simulink library "LibControllers"  (R2015b)
settings: Solver=ode45  SolverMode=SingleTasking  StartTime=0.0  StopTime=10.0  RelTol=1e-3
undefined symbols (not defined in the file or in its folder): accelCanon, adjustCoefficients, bw, depth, DiscIntNeverNeededParam, displCanon, forget, freq, initDispl, jerkCanon, kd, kdp, kf, ki, kp, maxAuthority, maxForce, nominFlow, p, R, ratedFlow, S, samplePeriod, T, velocCanon
undefined symbols (not defined in the file): fbkgen, fdp, fmax, fmin, gainRatio, interval, lagFreq, lagPhase, leadFreq, leadPhase, order, refabort, refgen, refsmooth, supplyPress, vmax, vmin
libraries: LibControllers x43, simulink x1
(part 2 of 2)

== system LibControllers/forward euler integrator with clipping ==
  inp : Inport
  Saturation : Saturate  UpperLimit=maxOutput  LowerLimit=minOutput
  Sum1 : Sum  Inputs=|++  SaturateOnIntegerOverflow=on  InputSameDT=on  OutDataTypeStr=Inherit: Same as first input
  T : Gain  Gain=samplePeriod
  Unit Delay : UnitDelay  SampleTime=-1
  Unit Delay1 : UnitDelay  InitialCondition=initialCondition  SampleTime=-1
  out : Outport
  wires:
  Saturation/1 -> Unit Delay1/1, out/1
  inp/1 -> Unit Delay/1
  Unit Delay/1 -> T/1
  Unit Delay1/1 -> Sum1/2
  Sum1/1 -> Saturation/1
  T/1 -> Sum1/1

== system LibControllers/generic controller ==
  cmd : Inport
  fbk : Inport  Port=2
  Sum : Sum  Inputs=|+-
  feedback polynomial : DiscreteFir  Coefficients=adjustCoefficients(S)  AccumDataTypeStr=Inherit: Same as product output
  feedforward polynomial : DiscreteFir  Coefficients=(T).'  AccumDataTypeStr=Inherit: Same as product output
  output scaling : Gain  Gain=k
  regression polynomial : DiscreteFilter  Denominator=R
  out : Outport
  wires:
  regression polynomial/1 -> output scaling/1
  Sum/1 -> regression polynomial/1
  feedforward polynomial/1 -> Sum/1
  feedback polynomial/1 -> Sum/2
  cmd/1 -> feedforward polynomial/1
  fbk/1 -> feedback polynomial/1
  output scaling/1 -> out/1

== system LibControllers/lag compensator ==
  inp : Inport
  Discrete Filter : DiscreteFilter  Numerator=b  Denominator=a
  out : Outport
  wires:
  Discrete Filter/1 -> out/1
  inp/1 -> Discrete Filter/1

== system LibControllers/lead compensator ==
  inp : Inport
  Discrete Filter : DiscreteFilter  Numerator=b  Denominator=a
  out : Outport
  wires:
  Discrete Filter/1 -> out/1
  inp/1 -> Discrete Filter/1

== system LibControllers/max//min cyclic fg ==
  Sum : Sum  Inputs=|++
  mean level : Constant  Value=mean
  shape : Constant  Value=shape
  sine wave : Sin  Amplitude=ampl  Frequency=2 * pi * freq  Phase=phase * pi/180  SampleTime=sourceSamplePeriod
  square wave : Subsystem  mask(Repeating table){ampl=ampl, freq=freq, phase=phase, samplePeriod=samplePeriod}
      mask prompts: ampl "Amplitude"; freq "Frequency (Hz)"; phase "Phase (deg)"; samplePeriod "Sample period (sec)"
      mask help: Output a repeating sequence of numbers specified in a table of time-value pairs. Values of time should be monotonically increasing.
      mask init:
      | % phase must be positive
      | while phase < 0
      | 	phase = phase + 360;
      | end
      mask Help: Repeats cycle given in table. Time values should be monotonically increasing.
  triangle wave : Subsystem  mask(Repeating table){ampl=ampl, freq=freq, phase=phase, samplePeriod=samplePeriod}
      mask prompts: ampl "Amplitude"; freq "Frequency (Hz)"; phase "Phase (deg)"; samplePeriod "Sample period (sec)"
      mask help: Output a repeating sequence of numbers specified in a table of time-value pairs. Values of time should be monotonically increasing.
      mask init:
      | % phase must be positive
      | while phase < 0
      | 	phase = phase + 360;
      | end
      mask Help: Repeats cycle given in table. Time values should be monotonically increasing.
  waveform selector : MultiPortSwitch
  out : Outport
  wires:
  mean level/1 -> Sum/2
  Sum/1 -> out/1
  shape/1 -> waveform selector/1
  square wave/1(out) -> waveform selector/2
  triangle wave/1(out) -> waveform selector/3
  sine wave/1 -> waveform selector/4
  waveform selector/1 -> Sum/1

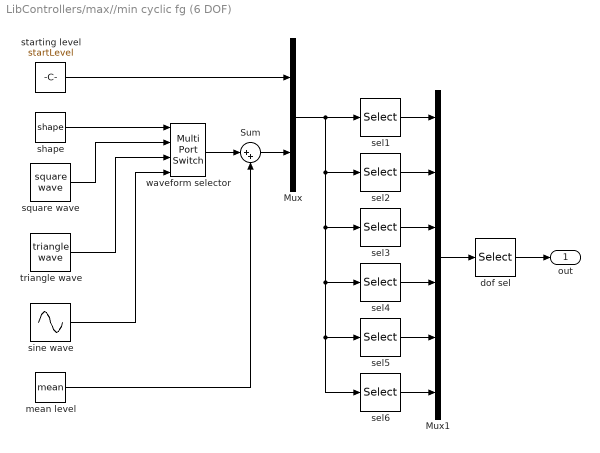
== system LibControllers/max//min cyclic fg (6 DOF) ==
  Mux : Mux  Inputs=2
  Mux1 : Mux  Inputs=6
  Sum : Sum  Inputs=|++
  dof sel : Selector  IndexOptions=Index vector (dialog)  Indices=dof  OutputSizes=1
  mean level : Constant  Value=mean
  sel1 : Selector  InputPortWidth=2  IndexOptions=Index vector (dialog)  Indices=(id==1)+1  OutputSizes=1
  sel2 : Selector  InputPortWidth=2  IndexOptions=Index vector (dialog)  Indices=(id==2)+1  OutputSizes=1
  sel3 : Selector  InputPortWidth=2  IndexOptions=Index vector (dialog)  Indices=(id==3)+1  OutputSizes=1
  sel4 : Selector  InputPortWidth=2  IndexOptions=Index vector (dialog)  Indices=(id==4)+1  OutputSizes=1
  sel5 : Selector  InputPortWidth=2  IndexOptions=Index vector (dialog)  Indices=(id==5)+1  OutputSizes=1
  sel6 : Selector  InputPortWidth=2  IndexOptions=Index vector (dialog)  Indices=(id==6)+1  OutputSizes=1
  shape : Constant  Value=shape
  sine wave : Sin  Amplitude=ampl  Frequency=2 * pi * freq  Phase=phase * pi/180  SampleTime=sourceSamplePeriod
  square wave : LibControllers/cyclic fg/square wave  SystemSampleTime=-1  ampl=ampl  freq=freq  phase=phase  samplePeriod=samplePeriod
  starting level : Constant  Value=startLevel
  triangle wave : LibControllers/cyclic fg/triangle wave  SystemSampleTime=-1  ampl=ampl  freq=freq  phase=phase  samplePeriod=samplePeriod
  waveform selector : MultiPortSwitch
  out : Outport
  wires:
  Sum/1 -> Mux/2
  waveform selector/1 -> Sum/1
  Mux1/1 -> dof sel/1
  mean level/1 -> Sum/2
  starting level/1 -> Mux/1
  sel1/1 -> Mux1/1
  sel2/1 -> Mux1/2
  sel3/1 -> Mux1/3
  sel4/1 -> Mux1/4
  sel5/1 -> Mux1/5
  sel6/1 -> Mux1/6
  Mux/1 -> sel2/1, sel3/1, sel4/1, sel5/1, sel6/1, sel1/1
  sine wave/1 -> waveform selector/4
  triangle wave/1 -> waveform selector/3
  square wave/1 -> waveform selector/2
  shape/1 -> waveform selector/1
  dof sel/1 -> out/1

== system LibControllers/notch filter ==
  inp : Inport
  Discrete Filter : DiscreteFilter  Numerator=b  Denominator=a
  out : Outport
  wires:
  Discrete Filter/1 -> out/1
  inp/1 -> Discrete Filter/1

== system LibControllers/pi controller ==
  cmd : Inport
  fbk : Inport  Port=2
  Sum : Sum  Inputs=|+-
  Sum1 : Sum  Inputs=|++
  egu to volts : Gain  Gain=10/maxUnits
  integrator with clipping : LibControllers/backward euler integrator with clipping  SystemSampleTime=-1  initialCondition=0  maxOutput=0.01*maxAuthority*maxUnits  minOutput=-0.01*maxAuthority*maxUnits  samplePeriod=samplePeriod
  ki : Gain  Gain=ki
  kp : Gain  Gain=kp
  out : Outport
  wires:
  Sum/1 -> kp/1, integrator with clipping/1
  cmd/1 -> Sum/1
  fbk/1 -> Sum/2
  kp/1 -> Sum1/1
  ki/1 -> Sum1/2
  integrator with clipping/1 -> ki/1
  Sum1/1 -> egu to volts/1
  egu to volts/1 -> out/1

== system LibControllers/pid controller ==
  cmd : Inport
  fbk : Inport  Port=2
  Sum : Sum  Inputs=|+-
  Sum1 : Sum  Inputs=++-
  Sum2 : Sum  Inputs=|++
  egu to volts : Gain  Gain=10/maxUnits
  fb break filter : Subsystem  mask(First-Order Lowpass Filter){freq=bw, samplePeriod=samplePeriod}
      mask prompts: freq "Cutoff frequency (Hz)"; samplePeriod "Sample period (sec)"
      mask init:
      | bwt = freq * samplePeriod;
      | if (bwt > 0.5*0.95) 
      | 	a = [1];
      | 	b = [1];
      | else	% first-order
      | 	c	 = 1 / tan(pi * bwt);
      | 	bwt2 = 1.0 / (pi * c);	% prewarp
      | 	a    = [1 -exp(-2*pi*bwt2)];
      | 	b	 = [1] * sum(a);
      | end
  fb derivative : LibControllers/euler derivative  SystemSampleTime=-1  initialCondition=0  samplePeriod=samplePeriod
  ff break filter : Subsystem  mask(First-Order Lowpass Filter){freq=bw, samplePeriod=samplePeriod}
      mask prompts: freq "Cutoff frequency (Hz)"; samplePeriod "Sample period (sec)"
      mask init:
      | bwt = freq * samplePeriod;
      | if (bwt > 0.5*0.95) 
      | 	a = [1];
      | 	b = [1];
      | else	% first-order
      | 	c	 = 1 / tan(pi * bwt);
      | 	bwt2 = 1.0 / (pi * c);	% prewarp
      | 	a    = [1 -exp(-2*pi*bwt2)];
      | 	b	 = [1] * sum(a);
      | end
  ff derivative : LibControllers/euler derivative  SystemSampleTime=-1  initialCondition=0  samplePeriod=samplePeriod
  integrator with clipping : LibControllers/backward euler integrator with clipping  SystemSampleTime=-1  initialCondition=0  maxOutput=0.01*maxAuthority*maxUnits  minOutput=-0.01*maxAuthority*maxUnits  samplePeriod=samplePeriod
  ki : Gain  Gain=ki
  ki1 : Gain  Gain=kd
  kp : Gain  Gain=kp
  kp1 : Gain  Gain=kf
  second-order butterworth lowpass filter : LibControllers/second-order butterworth lowpass filter  SystemSampleTime=-1  freq=bw  samplePeriod=samplePeriod
  out : Outport
  wires:
  egu to volts/1 -> out/1
  integrator with clipping/1 -> ki/1
  kp/1 -> Sum1/2
  kp1/1 -> Sum1/1
  fb break filter/1(out) -> ki1/1
  ff break filter/1(out) -> kp1/1
  second-order butterworth lowpass filter/1 -> Sum2/1
  Sum1/1 -> second-order butterworth lowpass filter/1
  ff derivative/1 -> ff break filter/1(inp)
  fbk/1 -> Sum/2, fb derivative/1
  cmd/1 -> Sum/1, ff derivative/1
  Sum/1 -> kp/1, integrator with clipping/1
  fb derivative/1 -> fb break filter/1(inp)
  ki1/1 -> Sum1/3
  Sum2/1 -> egu to volts/1
  ki/1 -> Sum2/2

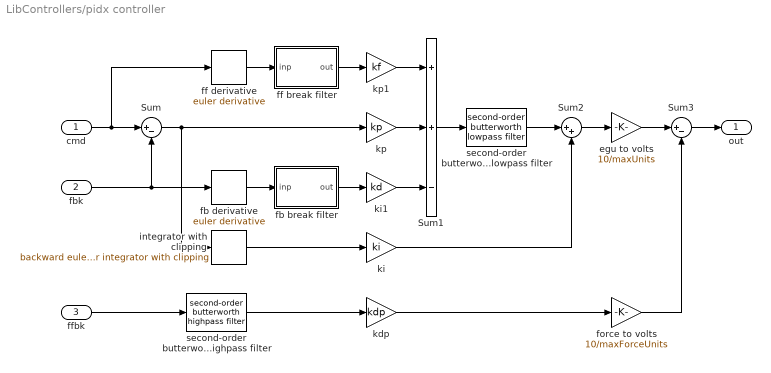
== system LibControllers/pidx controller ==
  cmd : Inport
  fbk : Inport  Port=2
  ffbk : Inport  Port=3
  Sum : Sum  Inputs=|+-
  Sum1 : Sum  Inputs=++-
  Sum2 : Sum  Inputs=|++
  Sum3 : Sum  Inputs=|+-
  egu to volts : Gain  Gain=10/maxUnits
  fb break filter : Subsystem  mask(First-Order Lowpass Filter){freq=bw, samplePeriod=samplePeriod}
      mask prompts: freq "Cutoff frequency (Hz)"; samplePeriod "Sample period (sec)"
      mask init:
      | bwt = freq * samplePeriod;
      | if (bwt > 0.5*0.95) 
      | 	a = [1];
      | 	b = [1];
      | else	% first-order
      | 	c	 = 1 / tan(pi * bwt);
      | 	bwt2 = 1.0 / (pi * c);	% prewarp
      | 	a    = [1 -exp(-2*pi*bwt2)];
      | 	b	 = [1] * sum(a);
      | end
  fb derivative : LibControllers/euler derivative  SystemSampleTime=-1  initialCondition=0  samplePeriod=samplePeriod
  ff break filter : Subsystem  mask(First-Order Lowpass Filter){freq=bw, samplePeriod=samplePeriod}
      mask prompts: freq "Cutoff frequency (Hz)"; samplePeriod "Sample period (sec)"
      mask init:
      | bwt = freq * samplePeriod;
      | if (bwt > 0.5*0.95) 
      | 	a = [1];
      | 	b = [1];
      | else	% first-order
      | 	c	 = 1 / tan(pi * bwt);
      | 	bwt2 = 1.0 / (pi * c);	% prewarp
      | 	a    = [1 -exp(-2*pi*bwt2)];
      | 	b	 = [1] * sum(a);
      | end
  ff derivative : LibControllers/euler derivative  SystemSampleTime=-1  initialCondition=0  samplePeriod=samplePeriod
  force to volts : Gain  Gain=10/maxForceUnits
  integrator with clipping : LibControllers/backward euler integrator with clipping  SystemSampleTime=-1  initialCondition=0  maxOutput=0.01*maxAuthority*maxUnits  minOutput=-0.01*maxAuthority*maxUnits  samplePeriod=samplePeriod
  kdp : Gain  Gain=kdp
  ki : Gain  Gain=ki
  ki1 : Gain  Gain=kd
  kp : Gain  Gain=kp
  kp1 : Gain  Gain=kf
  second-order butterworth highpass filter : LibControllers/second-order butterworth highpass filter  SystemSampleTime=-1  freq=fdp  samplePeriod=samplePeriod
  second-order butterworth lowpass filter : LibControllers/second-order butterworth lowpass filter  SystemSampleTime=-1  freq=bw  samplePeriod=samplePeriod
  out : Outport
  wires:
  ki/1 -> Sum2/2
  kdp/1 -> force to volts/1
  integrator with clipping/1 -> ki/1
  kp/1 -> Sum1/2
  kp1/1 -> Sum1/1
  fb break filter/1(out) -> ki1/1
  ff break filter/1(out) -> kp1/1
  second-order butterworth highpass filter/1 -> kdp/1
  second-order butterworth lowpass filter/1 -> Sum2/1
  Sum1/1 -> second-order butterworth lowpass filter/1
  ff derivative/1 -> ff break filter/1(inp)
  ffbk/1 -> second-order butterworth highpass filter/1
  fbk/1 -> Sum/2, fb derivative/1
  cmd/1 -> Sum/1, ff derivative/1
  Sum/1 -> kp/1, integrator with clipping/1
  fb derivative/1 -> fb break filter/1(inp)
  ki1/1 -> Sum1/3
  Sum3/1 -> out/1
  Sum2/1 -> egu to volts/1
  egu to volts/1 -> Sum3/1
  force to volts/1 -> Sum3/2

== system LibControllers/power observer ==
  veloc : Inport
  force : Inport  Port=2
  force polarity switch : Switch
  max force : Constant  Value=abs(max(fmax, eps))
  max veloc : Constant  Value=abs(max(vmax, eps))
  min force : Constant  Value=abs(min(fmin, eps))
  min veloc : Constant  Value=abs(min(vmin, eps))
  neg scale : Gain  Gain=100 / sqrt(2)
  normalization : Product  Inputs=*/
  normalization factor : Product  RndMeth=Zero
  pos scale : Gain  Gain=100 * 2 * sqrt(2)
  power calculation : Product  RndMeth=Zero
  power polarity switch : Switch
  velocity polarity switch : Switch
  power : Outport
  wires:
  veloc/1 -> power calculation/1, velocity polarity switch/2
  force/1 -> power calculation/2, force polarity switch/2
  power calculation/1 -> normalization/1
  min veloc/1 -> velocity polarity switch/3
  max veloc/1 -> velocity polarity switch/1
  max force/1 -> force polarity switch/1
  min force/1 -> force polarity switch/3
  velocity polarity switch/1 -> normalization factor/1
  force polarity switch/1 -> normalization factor/2
  normalization factor/1 -> normalization/2
  power polarity switch/1 -> power/1
  normalization/1 -> pos scale/1, power polarity switch/2, neg scale/1
  pos scale/1 -> power polarity switch/1
  neg scale/1 -> power polarity switch/3

== system LibControllers/ramp fg ==
  integrator with clipping : LibControllers/forward euler integrator with clipping  SystemSampleTime=-1  initialCondition=startLevel  maxOutput=max(startLevel, endLevel)  minOutput=min(startLevel, endLevel)  samplePeriod=samplePeriod
  ramp rate : Constant  Value=(endLevel - startLevel) / max(interval, samplePeriod)
  out : Outport
  wires:
  ramp rate/1 -> integrator with clipping/1
  integrator with clipping/1 -> out/1

== system LibControllers/rand fg ==
  Product : Product  RndMeth=Zero
  biquad group 1 : Subsystem  mask(Discrete Filter Group of Five Biquads){sos=sos(1:5,:)}
      mask prompts: sos "Second-order sections"
  biquad group 2 : Subsystem  mask(Discrete Filter Group of Five Biquads){sos=sos(6:10,:)}
      mask prompts: sos "Second-order sections"
  biquad group 3 : Subsystem  mask(Discrete Filter Group of Five Biquads){sos=sos(11:15,:)}
      mask prompts: sos "Second-order sections"
  gain : Gain  Gain=g
  span fg : LibControllers/ramp fg  SystemSampleTime=-1  startLevel=0  endLevel=1  interval=spanInterval  samplePeriod=samplePeriod
  uniform rand : UniformRandomNumber  Minimum=-peakAmpl  Maximum=peakAmpl  Seed=seed  SampleTime=sourceSamplePeriod
  out : Outport
  wires:
  biquad group 3/1(out) -> gain/1
  biquad group 2/1(out) -> biquad group 3/1(inp)
  biquad group 1/1(out) -> biquad group 2/1(inp)
  gain/1 -> Product/1
  uniform rand/1 -> biquad group 1/1(inp)
  Product/1 -> out/1
  span fg/1 -> Product/2

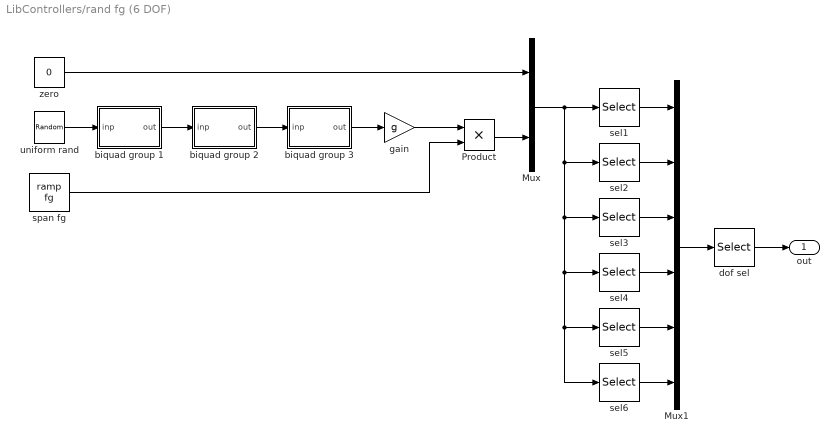
== system LibControllers/rand fg (6 DOF) ==
  Mux : Mux  Inputs=2
  Mux1 : Mux  Inputs=6
  Product : Product  RndMeth=Zero
  biquad group 1 : Subsystem  mask(Discrete Filter Group of Five Biquads){sos=sos(1:5,:)}
      mask prompts: sos "Second-order sections"
  biquad group 2 : Subsystem  mask(Discrete Filter Group of Five Biquads){sos=sos(6:10,:)}
      mask prompts: sos "Second-order sections"
  biquad group 3 : Subsystem  mask(Discrete Filter Group of Five Biquads){sos=sos(11:15,:)}
      mask prompts: sos "Second-order sections"
  dof sel : Selector  IndexOptions=Index vector (dialog)  Indices=dof  OutputSizes=1
  gain : Gain  Gain=g
  sel1 : Selector  InputPortWidth=2  IndexOptions=Index vector (dialog)  Indices=(id==1)+1  OutputSizes=1
  sel2 : Selector  InputPortWidth=2  IndexOptions=Index vector (dialog)  Indices=(id==2)+1  OutputSizes=1
  sel3 : Selector  InputPortWidth=2  IndexOptions=Index vector (dialog)  Indices=(id==3)+1  OutputSizes=1
  sel4 : Selector  InputPortWidth=2  IndexOptions=Index vector (dialog)  Indices=(id==4)+1  OutputSizes=1
  sel5 : Selector  InputPortWidth=2  IndexOptions=Index vector (dialog)  Indices=(id==5)+1  OutputSizes=1
  sel6 : Selector  InputPortWidth=2  IndexOptions=Index vector (dialog)  Indices=(id==6)+1  OutputSizes=1
  span fg : LibControllers/ramp fg  SystemSampleTime=-1  startLevel=0  endLevel=1  interval=spanInterval  samplePeriod=samplePeriod
  uniform rand : UniformRandomNumber  Minimum=-peakAmpl  Maximum=peakAmpl  Seed=seed  SampleTime=sourceSamplePeriod
  zero : Constant  Value=0
  out : Outport
  wires:
  Mux/1 -> sel2/1, sel3/1, sel4/1, sel5/1, sel6/1, sel1/1
  sel6/1 -> Mux1/6
  sel5/1 -> Mux1/5
  sel4/1 -> Mux1/4
  sel3/1 -> Mux1/3
  sel2/1 -> Mux1/2
  sel1/1 -> Mux1/1
  zero/1 -> Mux/1
  biquad group 3/1(out) -> gain/1
  biquad group 2/1(out) -> biquad group 3/1(inp)
  biquad group 1/1(out) -> biquad group 2/1(inp)
  uniform rand/1 -> biquad group 1/1(inp)
  Mux1/1 -> dof sel/1
  gain/1 -> Product/1
  span fg/1 -> Product/2
  Product/1 -> Mux/2
  dof sel/1 -> out/1

== system LibControllers/rate limiter ==
  inp : Inport
  integrator : LibControllers/forward euler integrator  SystemSampleTime=-1  initialCondition=initOutput  samplePeriod=1
  rate limit : Saturate  UpperLimit=rateMax * samplePeriod  LowerLimit=rateMin * samplePeriod
  rateCanon : Gain  Gain=rateCanon
  sum4 : Sum  Inputs=|+-
  out : Outport
  wires:
  rate limit/1 -> rateCanon/1
  inp/1 -> sum4/1
  sum4/1 -> rate limit/1
  integrator/1 -> out/1, sum4/2
  rateCanon/1 -> integrator/1

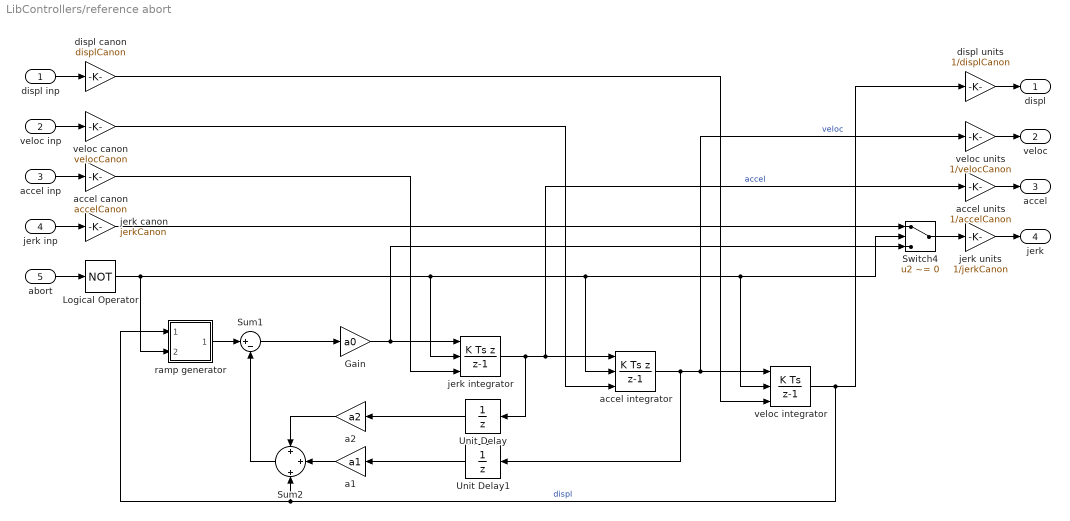
== system LibControllers/reference abort ==
  displ inp : Inport
  veloc inp : Inport  Port=2
  accel inp : Inport  Port=3
  jerk inp : Inport  Port=4
  abort : Inport  Port=5
  Gain : Gain  Gain=a0
  Logical Operator : Logic  Operator=NOT  AllPortsSameDT=off  OutDataTypeStr=boolean
  Sum1 : Sum  Inputs=|+-
  Sum2 : Sum  Inputs=+|+|+
  Switch4 : Switch  Criteria=u2 ~= 0  ZeroCross=off
  Unit Delay : UnitDelay  SampleTime=-1
  Unit Delay1 : UnitDelay  SampleTime=-1
  a1 : Gain  Gain=a1
  a2 : Gain  Gain=a2
  accel canon : Gain  Gain=accelCanon
  accel integrator : DiscreteIntegrator  IntegratorMethod=Integration: Backward Euler  ExternalReset=level  InitialConditionSource=external  SampleTime=-1  ICPrevOutput=DiscIntNeverNeededParam  ICPrevScaledInput=DiscIntNeverNeededParam
  accel units : Gain  Gain=1/accelCanon
  displ canon : Gain  Gain=displCanon
  displ units : Gain  Gain=1/displCanon
  jerk canon : Gain  Gain=jerkCanon
  jerk integrator : DiscreteIntegrator  IntegratorMethod=Integration: Backward Euler  ExternalReset=level  InitialConditionSource=external  SampleTime=-1  ICPrevOutput=DiscIntNeverNeededParam  ICPrevScaledInput=DiscIntNeverNeededParam
  jerk units : Gain  Gain=1/jerkCanon
  ramp generator : Subsystem
  veloc canon : Gain  Gain=velocCanon
  veloc integrator : DiscreteIntegrator  ExternalReset=level  InitialConditionSource=external  SampleTime=-1  ICPrevOutput=DiscIntNeverNeededParam  ICPrevScaledInput=DiscIntNeverNeededParam
  veloc units : Gain  Gain=1/velocCanon
  displ : Outport
  veloc : Outport  Port=2
  accel : Outport  Port=3
  jerk : Outport  Port=4
  wires:
  accel integrator/1 -> veloc units/1, veloc integrator/1, Unit Delay1/1  "veloc"
  Unit Delay1/1 -> a1/1
  Unit Delay/1 -> a2/1
  ramp generator/1(out) -> Sum1/1
  Sum2/1 -> Sum1/2
  Sum1/1 -> Gain/1
  Logical Operator/1 -> jerk integrator/2, accel integrator/2, veloc integrator/2, Switch4/2, ramp generator/2(abort)
  jerk canon/1 -> Switch4/1
  accel canon/1 -> jerk integrator/3
  veloc canon/1 -> accel integrator/3
  displ canon/1 -> veloc integrator/3
  abort/1 -> Logical Operator/1
  veloc integrator/1 -> Sum2/3, ramp generator/1(inp), displ units/1  "displ"
  jerk inp/1 -> jerk canon/1
  accel inp/1 -> accel canon/1
  veloc inp/1 -> veloc canon/1
  displ inp/1 -> displ canon/1
  jerk integrator/1 -> accel units/1, accel integrator/1, Unit Delay/1  "accel"
  Gain/1 -> Switch4/3, jerk integrator/1
  a2/1 -> Sum2/1
  accel units/1 -> accel/1
  veloc units/1 -> veloc/1
  displ units/1 -> displ/1
  jerk units/1 -> jerk/1
  Switch4/1 -> jerk units/1
  a1/1 -> Sum2/2

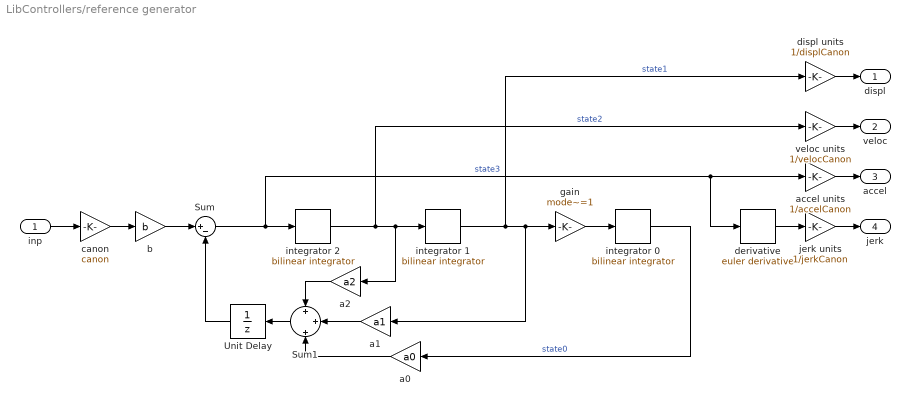
== system LibControllers/reference generator ==
  inp : Inport
  Sum : Sum  Inputs=|+-
  Sum1 : Sum  Inputs=+|+|+
  Unit Delay : UnitDelay  SampleTime=-1
  a0 : Gain  Gain=a0
  a1 : Gain  Gain=a1
  a2 : Gain  Gain=a2
  accel units : Gain  Gain=1/accelCanon
  b : Gain  Gain=b
  canon : Gain  Gain=canon
  derivative : LibControllers/euler derivative  SystemSampleTime=-1  initialCondition=0  samplePeriod=samplePeriod
  displ units : Gain  Gain=1/displCanon
  gain : Gain  Gain=mode~=1
  integrator 0 : LibControllers/bilinear integrator  SystemSampleTime=-1  initialCondition=0  samplePeriod=samplePeriod
  integrator 1 : LibControllers/bilinear integrator  SystemSampleTime=-1  initialCondition=0  samplePeriod=samplePeriod
  integrator 2 : LibControllers/bilinear integrator  SystemSampleTime=-1  initialCondition=0  samplePeriod=samplePeriod
  jerk units : Gain  Gain=1/jerkCanon
  veloc units : Gain  Gain=1/velocCanon
  displ : Outport
  veloc : Outport  Port=2
  accel : Outport  Port=3
  jerk : Outport  Port=4
  wires:
  integrator 2/1 -> a2/1, integrator 1/1, veloc units/1  "state2"
  integrator 1/1 -> a1/1, gain/1, displ units/1  "state1"
  Sum/1 -> accel units/1, derivative/1, integrator 2/1  "state3"
  b/1 -> Sum/1
  Sum1/1 -> Unit Delay/1
  a2/1 -> Sum1/1
  a1/1 -> Sum1/2
  a0/1 -> Sum1/3
  integrator 0/1 -> a0/1  "state0"
  inp/1 -> canon/1
  accel units/1 -> accel/1
  veloc units/1 -> veloc/1
  displ units/1 -> displ/1
  canon/1 -> b/1
  jerk units/1 -> jerk/1
  Unit Delay/1 -> Sum/2
  derivative/1 -> jerk units/1
  gain/1 -> integrator 0/1

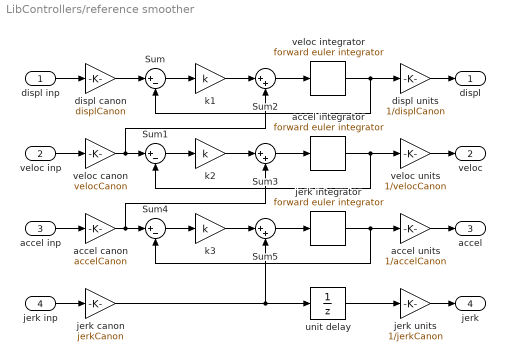
== system LibControllers/reference smoother ==
  displ inp : Inport
  veloc inp : Inport  Port=2
  accel inp : Inport  Port=3
  jerk inp : Inport  Port=4
  Sum : Sum  Inputs=|+-
  Sum1 : Sum  Inputs=|+-
  Sum2 : Sum  Inputs=|++
  Sum3 : Sum  Inputs=|++
  Sum4 : Sum  Inputs=|+-
  Sum5 : Sum  Inputs=|++
  accel canon : Gain  Gain=accelCanon
  accel integrator : LibControllers/forward euler integrator  SystemSampleTime=-1  initialCondition=0  samplePeriod=samplePeriod
  accel units : Gain  Gain=1/accelCanon
  displ canon : Gain  Gain=displCanon
  displ units : Gain  Gain=1/displCanon
  jerk canon : Gain  Gain=jerkCanon
  jerk integrator : LibControllers/forward euler integrator  SystemSampleTime=-1  initialCondition=0  samplePeriod=samplePeriod
  jerk units : Gain  Gain=1/jerkCanon
  k1 : Gain  Gain=k
  k2 : Gain  Gain=k
  k3 : Gain  Gain=k
  unit delay : UnitDelay  SampleTime=-1
  veloc canon : Gain  Gain=velocCanon
  veloc integrator : LibControllers/forward euler integrator  SystemSampleTime=-1  initialCondition=initDispl*displCanon  samplePeriod=samplePeriod
  veloc units : Gain  Gain=1/velocCanon
  displ : Outport
  veloc : Outport  Port=2
  accel : Outport  Port=3
  jerk : Outport  Port=4
  wires:
  displ units/1 -> displ/1
  veloc units/1 -> veloc/1
  displ inp/1 -> displ canon/1
  veloc inp/1 -> veloc canon/1
  displ canon/1 -> Sum/1
  veloc integrator/1 -> displ units/1, Sum/2
  Sum/1 -> k1/1
  k1/1 -> Sum2/1
  Sum2/1 -> veloc integrator/1
  accel units/1 -> accel/1
  accel inp/1 -> accel canon/1
  accel integrator/1 -> Sum1/2, veloc units/1
  Sum1/1 -> k2/1
  k2/1 -> Sum3/1
  Sum3/1 -> accel integrator/1
  veloc canon/1 -> Sum1/1, Sum2/2
  jerk units/1 -> jerk/1
  jerk inp/1 -> jerk canon/1
  jerk canon/1 -> unit delay/1, Sum5/2
  unit delay/1 -> jerk units/1
  jerk integrator/1 -> Sum4/2, accel units/1
  Sum4/1 -> k3/1
  k3/1 -> Sum5/1
  Sum5/1 -> jerk integrator/1
  accel canon/1 -> Sum4/1, Sum3/2

== system LibControllers/second-order butterworth highpass filter ==
  inp : Inport
  Discrete Filter : DiscreteFilter  Numerator=b  Denominator=a
  out : Outport
  wires:
  inp/1 -> Discrete Filter/1
  Discrete Filter/1 -> out/1

== system LibControllers/second-order butterworth lowpass filter ==
  inp : Inport
  Discrete Filter : DiscreteFilter  Numerator=b  Denominator=a
  out : Outport
  wires:
  inp/1 -> Discrete Filter/1
  Discrete Filter/1 -> out/1

== system LibControllers/second-order inverse lowpass filter ==
  inp : Inport
  discrete filter : DiscreteFilter  Numerator=b  Denominator=a
  out : Outport
  wires:
  discrete filter/1 -> out/1
  inp/1 -> discrete filter/1

== system LibControllers/second-order lowpass filter ==
  inp : Inport
  discrete filter : DiscreteFilter  Numerator=b  Denominator=a
  out : Outport
  wires:
  inp/1 -> discrete filter/1
  discrete filter/1 -> out/1

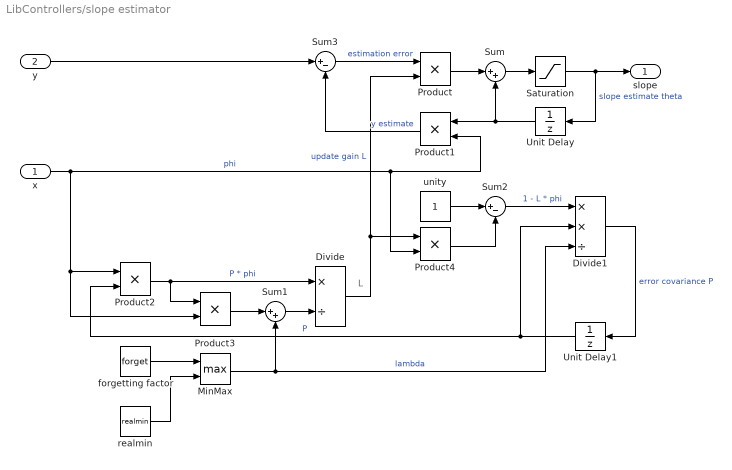
== system LibControllers/slope estimator ==
  note: L
  x : Inport
  y : Inport  Port=2
  Divide : Product  Inputs=*/
  Divide1 : Product  Inputs=**/
  MinMax : MinMax  Function=max  Inputs=2
  Product{,1..4} (5 alike) : Product  RndMeth=Zero
  Saturation : Saturate  UpperLimit=maxSlope  LowerLimit=minSlope
  Sum : Sum  Inputs=|++
  Sum1 : Sum  Inputs=|++
  Sum2 : Sum  Inputs=|+-
  Sum3 : Sum  Inputs=|+-
  Unit Delay : UnitDelay  InitialCondition=slope0  SampleTime=-1
  Unit Delay1 : UnitDelay  InitialCondition=errcov0  SampleTime=-1
  forgetting factor : Constant  Value=forget
  realmin : Constant  Value=realmin
  unity : Constant
  slope : Outport
  wires:
  Divide1/1 -> Unit Delay1/1  "error covariance P"
  Sum2/1 -> Divide1/1  "1 - L * phi"
  Product4/1 -> Sum2/2
  unity/1 -> Sum2/1
  Sum1/1 -> Divide/2
  Product3/1 -> Sum1/1
  MinMax/1 -> Divide1/3, Sum1/2  "lambda"
  Product2/1 -> Product3/1, Divide/1  "P * phi"
  Unit Delay1/1 -> Divide1/2, Product2/2  "P"
  Divide/1 -> Product/2, Product4/1  "update gain L"
  x/1 -> Product4/2, Product1/2, Product3/2, Product2/1  "phi"
  Product1/1 -> Sum3/2  "y estimate"
  y/1 -> Sum3/1
  Sum3/1 -> Product/1  "estimation error"
  Saturation/1 -> Unit Delay/1, slope/1  "slope estimate theta"
  Sum/1 -> Saturation/1
  Product/1 -> Sum/1
  Unit Delay/1 -> Product1/1, Sum/2
  forgetting factor/1 -> MinMax/1
  realmin/1 -> MinMax/2

== system LibControllers/sweep fg ==
  dwell : Inport
  Logical Operator : Logic  Operator=NOT  AllPortsSameDT=off  OutDataTypeStr=boolean
  Product : Product  RndMeth=Zero
  Product1 : Product  RndMeth=Zero
  Saturation : Saturate  UpperLimit=max(initialFreq, finalFreq)  LowerLimit=min(initialFreq, finalFreq)
  Sum1 : Sum  Inputs=|++  SaturateOnIntegerOverflow=on  InputSameDT=on  OutDataTypeStr=Inherit: Same as first input
  Sum2 : Sum  Inputs=|++  SaturateOnIntegerOverflow=on  InputSameDT=on  OutDataTypeStr=Inherit: Same as first input
  Unit Delay1 : UnitDelay  InitialCondition=initialFreq  SampleTime=-1
  ddf : Gain  Gain=ddf
  df : Constant  Value=df
  span fg : LibControllers/ramp fg  SystemSampleTime=-1  startLevel=0  endLevel=1  interval=spanInterval  samplePeriod=samplePeriod
  variable-frequency sine oscillator : LibControllers/variable-frequency sine oscillator  SystemSampleTime=-1  amplitude=ampl  samplePeriod=samplePeriod
  out : Outport
  freq : Outport  Port=2
  wires:
  variable-frequency sine oscillator/1 -> Product/1
  Product/1 -> out/1
  span fg/1 -> Product/2
  Sum1/1 -> Saturation/1
  Saturation/1 -> Unit Delay1/1, variable-frequency sine oscillator/1, freq/1
  Unit Delay1/1 -> ddf/1, Sum1/2
  ddf/1 -> Sum2/2
  df/1 -> Sum2/1
  Product1/1 -> Sum1/1
  Sum2/1 -> Product1/2
  dwell/1 -> Logical Operator/1
  Logical Operator/1 -> Product1/1

== system LibControllers/sweep fg (6 DOF) ==
  dwell : Inport
  Mux : Mux  Inputs=2
  Mux1 : Mux  Inputs=6
  Product2 : Product  RndMeth=Zero
  dof sel : Selector  IndexOptions=Index vector (dialog)  Indices=dof  OutputSizes=1
  sel1 : Selector  InputPortWidth=2  IndexOptions=Index vector (dialog)  Indices=(id==1)+1  OutputSizes=1
  sel2 : Selector  InputPortWidth=2  IndexOptions=Index vector (dialog)  Indices=(id==2)+1  OutputSizes=1
  sel3 : Selector  InputPortWidth=2  IndexOptions=Index vector (dialog)  Indices=(id==3)+1  OutputSizes=1
  sel4 : Selector  InputPortWidth=2  IndexOptions=Index vector (dialog)  Indices=(id==4)+1  OutputSizes=1
  sel5 : Selector  InputPortWidth=2  IndexOptions=Index vector (dialog)  Indices=(id==5)+1  OutputSizes=1
  sel6 : Selector  InputPortWidth=2  IndexOptions=Index vector (dialog)  Indices=(id==6)+1  OutputSizes=1
  span fg : LibControllers/ramp fg  SystemSampleTime=-1  startLevel=0  endLevel=1  interval=spanInterval  samplePeriod=samplePeriod
  sweep fg : Subsystem  mask(Sine Sweep Function Generator){ampl=ampl, initialFreq=initialFreq, finalFreq=finalFreq, sweepType=sweepType, rate=rate, spanInterval=spanInterval, samplePeriod=samplePeriod}
      mask prompts: ampl "Amplitude"; initialFreq "Initial frequency (Hz)"; finalFreq "Final frequency (Hz)"; sweepType "Sweep type (1: linear, 2: log)"; rate "Sweep rate (linear: Hz/sec, log: oct/min)"; spanInterval "Span interval (sec)"; samplePeriod "Sample period (sec)"
      mask init: same as LibControllers/sweep fg
  zero : Constant  Value=0
  out : Outport
  freq : Outport  Port=2
  wires:
  dwell/1 -> sweep fg/1(dwell)
  zero/1 -> Mux/1
  sel1/1 -> Mux1/1
  sel2/1 -> Mux1/2
  sel3/1 -> Mux1/3
  sel4/1 -> Mux1/4
  sel5/1 -> Mux1/5
  sel6/1 -> Mux1/6
  Mux/1 -> sel1/1, sel6/1, sel5/1, sel4/1, sel3/1, sel2/1
  Mux1/1 -> dof sel/1
  sweep fg/1(out) -> Product2/1
  Product2/1 -> Mux/2
  span fg/1 -> Product2/2
  dof sel/1 -> out/1
  sweep fg/2(freq) -> freq/1

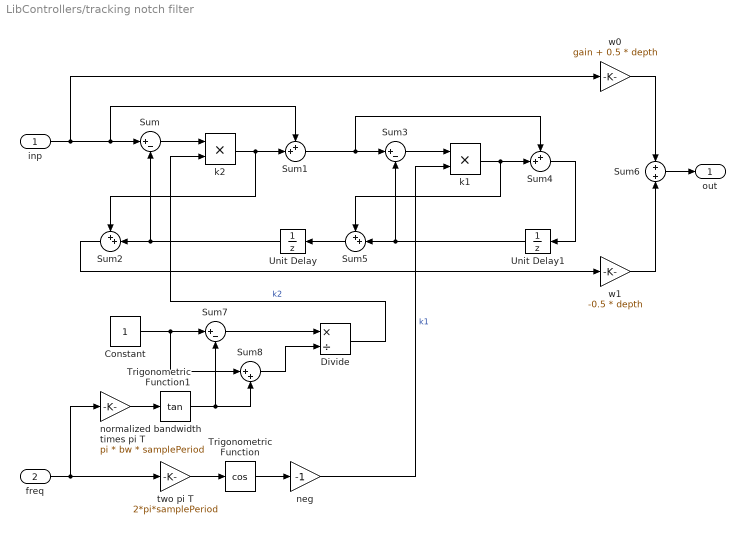
== system LibControllers/tracking notch filter ==
  inp : Inport
  freq : Inport  Port=2
  Constant : Constant
  Divide : Product  Inputs=*/
  Sum : Sum  Inputs=|+-
  Sum{1..2,4..5} (4 alike) : Sum  Inputs=++|
  Sum3 : Sum  Inputs=|+-
  Sum6 : Sum  Inputs=+|+
  Sum7 : Sum  Inputs=|+-
  Sum8 : Sum  Inputs=|++
  Trigonometric Function : Trigonometry  Operator=cos
  Trigonometric Function1 : Trigonometry  Operator=tan
  Unit Delay : UnitDelay  SampleTime=-1
  Unit Delay1 : UnitDelay  SampleTime=-1
  k1 : Product  RndMeth=Zero
  k2 : Product  RndMeth=Zero
  neg : Gain  Gain=-1
  normalized bandwidth times pi T : Gain  Gain=pi * bw * samplePeriod
  two pi T : Gain  Gain=2*pi*samplePeriod
  w0 : Gain  Gain=gain + 0.5 * depth
  w1 : Gain  Gain=-0.5 * depth
  out : Outport
  wires:
  Divide/1 -> k2/2  "k2"
  Trigonometric Function1/1 -> Sum8/2, Sum7/2
  Sum8/1 -> Divide/2
  normalized bandwidth times pi T/1 -> Trigonometric Function1/1
  Sum2/1 -> w1/1
  Sum6/1 -> out/1
  w1/1 -> Sum6/2
  w0/1 -> Sum6/1
  Sum4/1 -> Unit Delay1/1
  Sum5/1 -> Unit Delay/1
  Unit Delay1/1 -> Sum3/2, Sum5/2
  Sum3/1 -> k1/1
  Sum1/1 -> Sum3/1, Sum4/1
  Unit Delay/1 -> Sum2/2, Sum/2
  k2/1 -> Sum1/2, Sum2/1
  Sum/1 -> k2/1
  inp/1 -> w0/1, Sum1/1, Sum/1
  k1/1 -> Sum4/2, Sum5/1
  freq/1 -> normalized bandwidth times pi T/1, two pi T/1
  two pi T/1 -> Trigonometric Function/1
  Trigonometric Function/1 -> neg/1
  neg/1 -> k1/2  "k1"
  Constant/1 -> Sum8/1, Sum7/1
  Sum7/1 -> Divide/1

== system LibControllers/tvc controller ==
  ref : Inport
  displ fbk : Inport  Port=2
  accel fbk : Inport  Port=3
  force fbk : Inport  Port=4
  sel{1,5..7} (4 alike) : Selector  IndexOptions=Index vector (dialog)  Indices=p.id  OutputSizes=1
  three-variable controller : Subsystem
  out : Outport
  testpoints : Outport  Port=2
  wires:
  ref/1 -> sel1/1
  accel fbk/1 -> sel6/1
  displ fbk/1 -> sel5/1
  force fbk/1 -> sel7/1
  sel5/1 -> three-variable controller/2(displ fbk)
  sel6/1 -> three-variable controller/3(accel fbk)
  sel7/1 -> three-variable controller/4(force fbk)
  three-variable controller/1(out) -> out/1
  sel1/1 -> three-variable controller/1(ref)
  three-variable controller/2(testpoints) -> testpoints/1

== system LibControllers/variable-frequency sine oscillator ==
  freq : Inport
  Hz to rad/s : Gain  Gain=2*pi
  Sine Wave Function : Sin  TimeSource=Use external signal  Amplitude=amplitude  SampleTime=0
  Sum1 : Sum  Inputs=|++  SaturateOnIntegerOverflow=on  InputSameDT=on  OutDataTypeStr=Inherit: Same as first input
  T : Gain  Gain=samplePeriod
  Unit Delay1 : UnitDelay  SampleTime=-1
  phase wrap : Subsystem
  out : Outport
  wires:
  phase wrap/1(out) -> Unit Delay1/1, Sine Wave Function/1
  Sum1/1 -> phase wrap/1(inp)
  Unit Delay1/1 -> Sum1/2
  T/1 -> Sum1/1
  Hz to rad/s/1 -> T/1
  Sine Wave Function/1 -> out/1
  freq/1 -> Hz to rad/s/1

== system LibControllers/butterworth lowpass filter/biquad group 1 ==
  inp : Inport
  biquad 1 : DiscreteFilter  Numerator=sos(1,1:3)  Denominator=sos(1,4:6)
  biquad 2 : DiscreteFilter  Numerator=sos(2,1:3)  Denominator=sos(2,4:6)
  biquad 3 : DiscreteFilter  Numerator=sos(3,1:3)  Denominator=sos(3,4:6)
  biquad 4 : DiscreteFilter  Numerator=sos(4,1:3)  Denominator=sos(4,4:6)
  biquad 5 : DiscreteFilter  Numerator=sos(5,1:3)  Denominator=sos(5,4:6)
  out : Outport
  wires:
  inp/1 -> biquad 1/1
  biquad 1/1 -> biquad 2/1
  biquad 2/1 -> biquad 3/1
  biquad 3/1 -> biquad 4/1
  biquad 4/1 -> biquad 5/1
  biquad 5/1 -> out/1

== system LibControllers/butterworth lowpass filter/biquad group 2 ==
  inp : Inport
  biquad 1 : DiscreteFilter  Numerator=sos(1,1:3)  Denominator=sos(1,4:6)
  biquad 2 : DiscreteFilter  Numerator=sos(2,1:3)  Denominator=sos(2,4:6)
  biquad 3 : DiscreteFilter  Numerator=sos(3,1:3)  Denominator=sos(3,4:6)
  biquad 4 : DiscreteFilter  Numerator=sos(4,1:3)  Denominator=sos(4,4:6)
  biquad 5 : DiscreteFilter  Numerator=sos(5,1:3)  Denominator=sos(5,4:6)
  out : Outport
  wires:
  biquad 5/1 -> out/1
  biquad 4/1 -> biquad 5/1
  biquad 3/1 -> biquad 4/1
  biquad 2/1 -> biquad 3/1
  biquad 1/1 -> biquad 2/1
  inp/1 -> biquad 1/1

== system LibControllers/butterworth lowpass filter/biquad group 3 ==
  inp : Inport
  biquad 1 : DiscreteFilter  Numerator=sos(1,1:3)  Denominator=sos(1,4:6)
  biquad 2 : DiscreteFilter  Numerator=sos(2,1:3)  Denominator=sos(2,4:6)
  biquad 3 : DiscreteFilter  Numerator=sos(3,1:3)  Denominator=sos(3,4:6)
  biquad 4 : DiscreteFilter  Numerator=sos(4,1:3)  Denominator=sos(4,4:6)
  biquad 5 : DiscreteFilter  Numerator=sos(5,1:3)  Denominator=sos(5,4:6)
  out : Outport
  wires:
  inp/1 -> biquad 1/1
  biquad 1/1 -> biquad 2/1
  biquad 2/1 -> biquad 3/1
  biquad 3/1 -> biquad 4/1
  biquad 4/1 -> biquad 5/1
  biquad 5/1 -> out/1

== system LibControllers/cyclic fg/square wave ==
  Lookup Table : Lookup  InputValues=[0 0.5/freq 1/freq]  Table=[-ampl ampl -ampl]  LookUpMeth=Use Input Nearest
  Sum1 : Sum  Inputs=|++  SaturateOnIntegerOverflow=on  InputSameDT=on  OutDataTypeStr=Inherit: Same as first input
  T : Constant  Value=samplePeriod
  Unit Delay1 : UnitDelay  InitialCondition=((phase+90)/360) / freq  SampleTime=-1
  period : Constant  Value=1/freq
  remainder : Math  Operator=rem  SaturateOnIntegerOverflow=on
  out : Outport
  wires:
  Sum1/1 -> Unit Delay1/1, remainder/1
  Unit Delay1/1 -> Sum1/2
  T/1 -> Sum1/1
  Lookup Table/1 -> out/1
  period/1 -> remainder/2
  remainder/1 -> Lookup Table/1

== system LibControllers/cyclic fg/triangle wave ==
  Lookup Table : Lookup  InputValues=[0 0.5/freq 1/freq]  Table=[-ampl ampl -ampl]
  Sum1 : Sum  Inputs=|++  SaturateOnIntegerOverflow=on  InputSameDT=on  OutDataTypeStr=Inherit: Same as first input
  T : Constant  Value=samplePeriod
  Unit Delay1 : UnitDelay  InitialCondition=((phase+90)/360) / freq  SampleTime=-1
  period : Constant  Value=1/freq
  remainder : Math  Operator=rem  SaturateOnIntegerOverflow=on
  out : Outport
  wires:
  remainder/1 -> Lookup Table/1
  period/1 -> remainder/2
  Lookup Table/1 -> out/1
  T/1 -> Sum1/1
  Unit Delay1/1 -> Sum1/2
  Sum1/1 -> remainder/1, Unit Delay1/1

== system LibControllers/max//min cyclic fg/square wave ==
  Lookup Table : Lookup  InputValues=[0 0.5/freq 1/freq]  Table=[-ampl ampl -ampl]  LookUpMeth=Use Input Nearest
  Sum1 : Sum  Inputs=|++  SaturateOnIntegerOverflow=on  InputSameDT=on  OutDataTypeStr=Inherit: Same as first input
  T : Constant  Value=samplePeriod
  Unit Delay1 : UnitDelay  InitialCondition=((phase+90)/360) / freq  SampleTime=-1
  period : Constant  Value=1/freq
  remainder : Math  Operator=rem  SaturateOnIntegerOverflow=on
  out : Outport
  wires:
  remainder/1 -> Lookup Table/1
  period/1 -> remainder/2
  Lookup Table/1 -> out/1
  T/1 -> Sum1/1
  Unit Delay1/1 -> Sum1/2
  Sum1/1 -> remainder/1, Unit Delay1/1

== system LibControllers/max//min cyclic fg/triangle wave ==
  Lookup Table : Lookup  InputValues=[0 0.5/freq 1/freq]  Table=[-ampl ampl -ampl]
  Sum1 : Sum  Inputs=|++  SaturateOnIntegerOverflow=on  InputSameDT=on  OutDataTypeStr=Inherit: Same as first input
  T : Constant  Value=samplePeriod
  Unit Delay1 : UnitDelay  InitialCondition=((phase+90)/360) / freq  SampleTime=-1
  period : Constant  Value=1/freq
  remainder : Math  Operator=rem  SaturateOnIntegerOverflow=on
  out : Outport
  wires:
  Sum1/1 -> Unit Delay1/1, remainder/1
  Unit Delay1/1 -> Sum1/2
  T/1 -> Sum1/1
  Lookup Table/1 -> out/1
  period/1 -> remainder/2
  remainder/1 -> Lookup Table/1

== system LibControllers/pid controller/fb break filter ==
  inp : Inport
  Discrete Filter : DiscreteFilter  Numerator=b  Denominator=a
  out : Outport
  wires:
  Discrete Filter/1 -> out/1
  inp/1 -> Discrete Filter/1

== system LibControllers/pid controller/ff break filter ==
  inp : Inport
  Discrete Filter : DiscreteFilter  Numerator=b  Denominator=a
  out : Outport
  wires:
  inp/1 -> Discrete Filter/1
  Discrete Filter/1 -> out/1

== system LibControllers/pidx controller/fb break filter ==
  inp : Inport
  Discrete Filter : DiscreteFilter  Numerator=b  Denominator=a
  out : Outport
  wires:
  inp/1 -> Discrete Filter/1
  Discrete Filter/1 -> out/1

== system LibControllers/pidx controller/ff break filter ==
  inp : Inport
  Discrete Filter : DiscreteFilter  Numerator=b  Denominator=a
  out : Outport
  wires:
  Discrete Filter/1 -> out/1
  inp/1 -> Discrete Filter/1

== system LibControllers/rand fg/biquad group 1 ==
  inp : Inport
  biquad 1 : DiscreteFilter  Numerator=sos(1,1:3)  Denominator=sos(1,4:6)
  biquad 2 : DiscreteFilter  Numerator=sos(2,1:3)  Denominator=sos(2,4:6)
  biquad 3 : DiscreteFilter  Numerator=sos(3,1:3)  Denominator=sos(3,4:6)
  biquad 4 : DiscreteFilter  Numerator=sos(4,1:3)  Denominator=sos(4,4:6)
  biquad 5 : DiscreteFilter  Numerator=sos(5,1:3)  Denominator=sos(5,4:6)
  out : Outport
  wires:
  biquad 5/1 -> out/1
  biquad 4/1 -> biquad 5/1
  biquad 3/1 -> biquad 4/1
  biquad 2/1 -> biquad 3/1
  biquad 1/1 -> biquad 2/1
  inp/1 -> biquad 1/1

== system LibControllers/rand fg/biquad group 2 ==
  inp : Inport
  biquad 1 : DiscreteFilter  Numerator=sos(1,1:3)  Denominator=sos(1,4:6)
  biquad 2 : DiscreteFilter  Numerator=sos(2,1:3)  Denominator=sos(2,4:6)
  biquad 3 : DiscreteFilter  Numerator=sos(3,1:3)  Denominator=sos(3,4:6)
  biquad 4 : DiscreteFilter  Numerator=sos(4,1:3)  Denominator=sos(4,4:6)
  biquad 5 : DiscreteFilter  Numerator=sos(5,1:3)  Denominator=sos(5,4:6)
  out : Outport
  wires:
  inp/1 -> biquad 1/1
  biquad 1/1 -> biquad 2/1
  biquad 2/1 -> biquad 3/1
  biquad 3/1 -> biquad 4/1
  biquad 4/1 -> biquad 5/1
  biquad 5/1 -> out/1

== system LibControllers/rand fg/biquad group 3 ==
  inp : Inport
  biquad 1 : DiscreteFilter  Numerator=sos(1,1:3)  Denominator=sos(1,4:6)
  biquad 2 : DiscreteFilter  Numerator=sos(2,1:3)  Denominator=sos(2,4:6)
  biquad 3 : DiscreteFilter  Numerator=sos(3,1:3)  Denominator=sos(3,4:6)
  biquad 4 : DiscreteFilter  Numerator=sos(4,1:3)  Denominator=sos(4,4:6)
  biquad 5 : DiscreteFilter  Numerator=sos(5,1:3)  Denominator=sos(5,4:6)
  out : Outport
  wires:
  biquad 5/1 -> out/1
  biquad 4/1 -> biquad 5/1
  biquad 3/1 -> biquad 4/1
  biquad 2/1 -> biquad 3/1
  biquad 1/1 -> biquad 2/1
  inp/1 -> biquad 1/1

== system LibControllers/rand fg (6 DOF)/biquad group 1 ==
  inp : Inport
  biquad 1 : DiscreteFilter  Numerator=sos(1,1:3)  Denominator=sos(1,4:6)
  biquad 2 : DiscreteFilter  Numerator=sos(2,1:3)  Denominator=sos(2,4:6)
  biquad 3 : DiscreteFilter  Numerator=sos(3,1:3)  Denominator=sos(3,4:6)
  biquad 4 : DiscreteFilter  Numerator=sos(4,1:3)  Denominator=sos(4,4:6)
  biquad 5 : DiscreteFilter  Numerator=sos(5,1:3)  Denominator=sos(5,4:6)
  out : Outport
  wires:
  biquad 5/1 -> out/1
  biquad 4/1 -> biquad 5/1
  biquad 3/1 -> biquad 4/1
  biquad 2/1 -> biquad 3/1
  biquad 1/1 -> biquad 2/1
  inp/1 -> biquad 1/1

== system LibControllers/rand fg (6 DOF)/biquad group 2 ==
  inp : Inport
  biquad 1 : DiscreteFilter  Numerator=sos(1,1:3)  Denominator=sos(1,4:6)
  biquad 2 : DiscreteFilter  Numerator=sos(2,1:3)  Denominator=sos(2,4:6)
  biquad 3 : DiscreteFilter  Numerator=sos(3,1:3)  Denominator=sos(3,4:6)
  biquad 4 : DiscreteFilter  Numerator=sos(4,1:3)  Denominator=sos(4,4:6)
  biquad 5 : DiscreteFilter  Numerator=sos(5,1:3)  Denominator=sos(5,4:6)
  out : Outport
  wires:
  inp/1 -> biquad 1/1
  biquad 1/1 -> biquad 2/1
  biquad 2/1 -> biquad 3/1
  biquad 3/1 -> biquad 4/1
  biquad 4/1 -> biquad 5/1
  biquad 5/1 -> out/1

== system LibControllers/rand fg (6 DOF)/biquad group 3 ==
  inp : Inport
  biquad 1 : DiscreteFilter  Numerator=sos(1,1:3)  Denominator=sos(1,4:6)
  biquad 2 : DiscreteFilter  Numerator=sos(2,1:3)  Denominator=sos(2,4:6)
  biquad 3 : DiscreteFilter  Numerator=sos(3,1:3)  Denominator=sos(3,4:6)
  biquad 4 : DiscreteFilter  Numerator=sos(4,1:3)  Denominator=sos(4,4:6)
  biquad 5 : DiscreteFilter  Numerator=sos(5,1:3)  Denominator=sos(5,4:6)
  out : Outport
  wires:
  biquad 5/1 -> out/1
  biquad 4/1 -> biquad 5/1
  biquad 3/1 -> biquad 4/1
  biquad 2/1 -> biquad 3/1
  biquad 1/1 -> biquad 2/1
  inp/1 -> biquad 1/1

== system LibControllers/reference abort/ramp generator ==
  inp : Inport
  abort : Inport  Port=2
  1/T : Gain  Gain=1/samplePeriod
  Compare To Constant : simulink/Logic and Bit Operations/Compare To Constant  SystemSampleTime=-1  relop===  const=2  LogicOutDataTypeMode=uint8  ZeroCross=off
  Constant1 : Constant  Value=0
  Constant2 : Constant  Value=mode
  Logical Operator : Logic  Operator=OR  AllPortsSameDT=off  OutDataTypeStr=boolean
  Multiport Switch : MultiPortSwitch  DataPortOrder=Zero-based contiguous  zeroidx=on
  ramp integrator : DiscreteIntegrator  ExternalReset=level  InitialConditionSource=external  SampleTime=-1  ICPrevOutput=DiscIntNeverNeededParam  ICPrevScaledInput=DiscIntNeverNeededParam
  ramp limit : Saturate  UpperLimit=rate*velocCanon  LowerLimit=-rate*velocCanon
  sample/hold : Subsystem  TreatAsAtomicUnit=on
  sum4 : Sum  Inputs=|+-
  out : Outport
  wires:
  Logical Operator/1 -> sample/hold/Enable, ramp integrator/2
  abort/1 -> Logical Operator/1
  Compare To Constant/1 -> Logical Operator/2
  Constant2/1 -> Compare To Constant/1, Multiport Switch/1
  sample/hold/1(out) -> sum4/1  "target"
  Multiport Switch/1 -> sample/hold/1(inp)
  inp/1 -> ramp integrator/3, Multiport Switch/4, Multiport Switch/3
  Constant1/1 -> Multiport Switch/2
  ramp limit/1 -> ramp integrator/1
  1/T/1 -> ramp limit/1
  sum4/1 -> 1/T/1
  ramp integrator/1 -> out/1, sum4/2

== system LibControllers/sweep fg (6 DOF)/sweep fg ==
  dwell : Inport
  Logical Operator : Logic  Operator=NOT  AllPortsSameDT=off  OutDataTypeStr=boolean
  Product : Product  RndMeth=Zero
  Product1 : Product  RndMeth=Zero
  Saturation : Saturate  UpperLimit=max(initialFreq, finalFreq)  LowerLimit=min(initialFreq, finalFreq)
  Sum1 : Sum  Inputs=|++  SaturateOnIntegerOverflow=on  InputSameDT=on  OutDataTypeStr=Inherit: Same as first input
  Sum2 : Sum  Inputs=|++  SaturateOnIntegerOverflow=on  InputSameDT=on  OutDataTypeStr=Inherit: Same as first input
  Unit Delay1 : UnitDelay  InitialCondition=initialFreq  SampleTime=-1
  ddf : Gain  Gain=ddf
  df : Constant  Value=df
  span fg : LibControllers/ramp fg  SystemSampleTime=-1  startLevel=0  endLevel=1  interval=spanInterval  samplePeriod=samplePeriod
  variable-frequency sine oscillator : LibControllers/variable-frequency sine oscillator  SystemSampleTime=-1  amplitude=ampl  samplePeriod=samplePeriod
  out : Outport
  freq : Outport  Port=2
  wires:
  variable-frequency sine oscillator/1 -> Product/1
  Product/1 -> out/1
  span fg/1 -> Product/2
  Sum1/1 -> Saturation/1
  Saturation/1 -> Unit Delay1/1, variable-frequency sine oscillator/1, freq/1
  Unit Delay1/1 -> ddf/1, Sum1/2
  ddf/1 -> Sum2/2
  df/1 -> Sum2/1
  Product1/1 -> Sum1/1
  Sum2/1 -> Product1/2
  dwell/1 -> Logical Operator/1
  Logical Operator/1 -> Product1/1

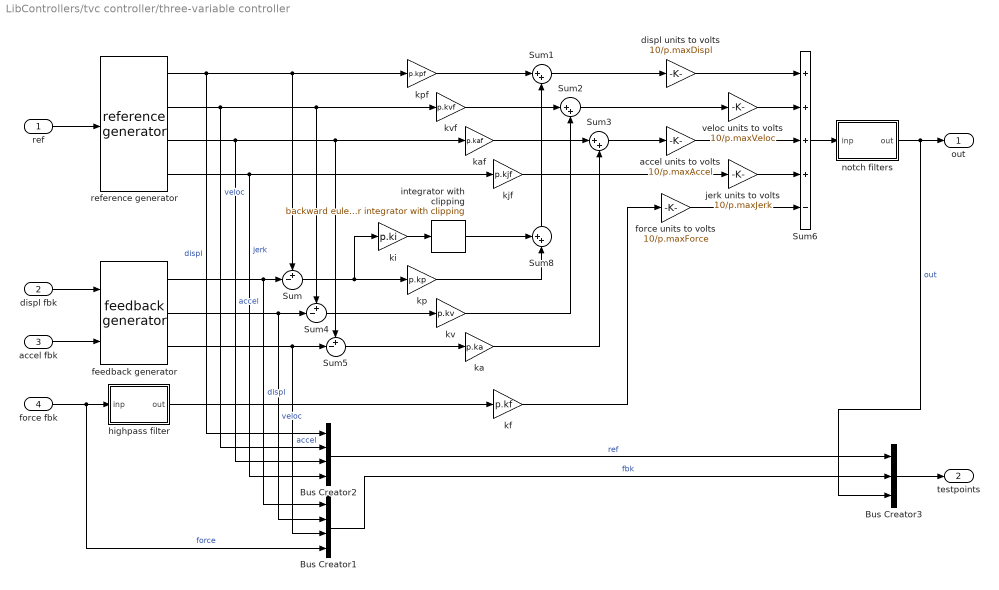
== system LibControllers/tvc controller/three-variable controller ==
  ref : Inport
  displ fbk : Inport  Port=2
  accel fbk : Inport  Port=3
  force fbk : Inport  Port=4
  Bus Creator1 : BusCreator  Inputs=4
  Bus Creator2 : BusCreator  Inputs=4
  Bus Creator3 : BusCreator  Inputs=3
  Sum : Sum  Inputs=+-|
  Sum1 : Sum  Inputs=|++
  Sum2 : Sum  Inputs=|++
  Sum3 : Sum  Inputs=|++
  Sum4 : Sum  Inputs=+-|
  Sum5 : Sum  Inputs=+-|
  Sum6 : Sum  Inputs=++++-
  Sum8 : Sum  Inputs=++|
  accel units to volts : Gain  Gain=10/p.maxAccel
  displ units to volts : Gain  Gain=10/p.maxDispl
  feedback generator : LibControllers/feedback generator  SystemSampleTime=-1  freq=p.fbkgen.freq  damp=p.fbkgen.damp  direct=p.fbkgen.direct  displCanon=p.displCanon  velocCanon=p.velocCanon  accelCanon=p.accelCanon  initDispl=p.initDispl  samplePeriod=samplePeriod
  force units to volts : Gain  Gain=10/p.maxForce
  highpass filter : Subsystem  mask{freq=p.hpfFreq, samplePeriod=samplePeriod}
      mask prompts: freq "Cut-in frequency (Hz)"; samplePeriod "Sample period (sec)"
      mask init: same as LibControllers/second-order butterworth highpass filter
  integrator with clipping : LibControllers/backward euler integrator with clipping  SystemSampleTime=-1  initialCondition=0  maxOutput=p.maxDispl*p.authority*0.01  minOutput=-p.maxDispl*p.authority*0.01  samplePeriod=samplePeriod
  jerk units to volts : Gain  Gain=10/p.maxJerk
  ka : Gain  Gain=p.ka
  kaf : Gain  Gain=p.kaf
  kf : Gain  Gain=p.kf
  ki : Gain  Gain=p.ki
  kjf : Gain  Gain=p.kjf
  kp : Gain  Gain=p.kp
  kpf : Gain  Gain=p.kpf
  kv : Gain  Gain=p.kv
  kvf : Gain  Gain=p.kvf
  notch filters : Subsystem
  reference generator : LibControllers/reference generator  SystemSampleTime=-1  mode=p.refgen.mode  freqHP=p.refgen.hpfFreq  freqLP=p.refgen.lpfFreq  displCanon=p.displCanon  velocCanon=p.velocCanon  accelCanon=p.accelCanon  jerkCanon=p.jerkCanon  samplePeriod=samplePeriod
  veloc units to volts : Gain  Gain=10/p.maxVeloc
  out : Outport
  testpoints : Outport  Port=2
  wires:
  Bus Creator3/1 -> testpoints/1
  Bus Creator1/1 -> Bus Creator3/2  "fbk"
  Bus Creator2/1 -> Bus Creator3/1  "ref"
  reference generator/1 -> Bus Creator2/1, Sum/1, kpf/1  "displ"
  ref/1 -> reference generator/1
  reference generator/4 -> Bus Creator2/4, kjf/1  "jerk"
  reference generator/3 -> Bus Creator2/3, kaf/1, Sum5/1  "accel"
  reference generator/2 -> Bus Creator2/2, kvf/1, Sum4/1  "veloc"
  kf/1 -> force units to volts/1
  highpass filter/1(out) -> kf/1
  feedback generator/1 -> Bus Creator1/1, Sum/2  "displ"
  Sum/1 -> kp/1, ki/1
  kpf/1 -> Sum1/1
  Sum1/1 -> displ units to volts/1
  feedback generator/2 -> Bus Creator1/2, Sum4/2  "veloc"
  kvf/1 -> Sum2/1
  kv/1 -> Sum2/2
  kaf/1 -> Sum3/1
  feedback generator/3 -> Bus Creator1/3, Sum5/2  "accel"
  ka/1 -> Sum3/2
  kjf/1 -> jerk units to volts/1
  displ units to volts/1 -> Sum6/1
  jerk units to volts/1 -> Sum6/4
  force units to volts/1 -> Sum6/5
  ki/1 -> integrator with clipping/1
  displ fbk/1 -> feedback generator/1
  accel fbk/1 -> feedback generator/2
  force fbk/1 -> Bus Creator1/4, highpass filter/1(inp)  "force"
  notch filters/1(out) -> Bus Creator3/3, out/1  "out"
  Sum3/1 -> accel units to volts/1
  accel units to volts/1 -> Sum6/3
  Sum2/1 -> veloc units to volts/1
  veloc units to volts/1 -> Sum6/2
  Sum4/1 -> kv/1
  Sum5/1 -> ka/1
  integrator with clipping/1 -> Sum8/1
  kp/1 -> Sum8/2
  Sum8/1 -> Sum1/2
  Sum6/1 -> notch filters/1(inp)

== system LibControllers/variable-frequency sine oscillator/phase wrap ==
  inp : Inport
  Constant : Constant  Value=2*pi
  Relational Operator : RelationalOperator  Operator=>  OutDataTypeStr=boolean
  Sum : Sum  Inputs=|+-
  Switch : Switch  Criteria=u2 ~= 0
  out : Outport
  wires:
  Constant/1 -> Sum/2, Relational Operator/2
  Sum/1 -> Switch/1
  inp/1 -> Relational Operator/1, Switch/3, Sum/1
  Switch/1 -> out/1
  Relational Operator/1 -> Switch/2

== system LibControllers/reference abort/ramp generator/sample//hold ==
  inp : Inport
  Enable : EnablePort
  out : Outport
  wires:
  inp/1 -> out/1

== system LibControllers/tvc controller/three-variable controller/highpass filter ==
  inp : Inport
  Discrete Filter : DiscreteFilter  Numerator=b  Denominator=a
  out : Outport
  wires:
  inp/1 -> Discrete Filter/1
  Discrete Filter/1 -> out/1

== system LibControllers/tvc controller/three-variable controller/notch filters ==
  inp : Inport
  notch filter 1 : LibControllers/notch filter  SystemSampleTime=-1  freq=p.notch(1).freq  bw=p.notch(1).bw  depth=p.notch(1).depth  gain=1  samplePeriod=samplePeriod
  notch filter 2 : LibControllers/notch filter  SystemSampleTime=-1  freq=p.notch(2).freq  bw=p.notch(2).bw  depth=p.notch(2).depth  gain=1  samplePeriod=samplePeriod
  notch filter 3 : LibControllers/notch filter  SystemSampleTime=-1  freq=p.notch(3).freq  bw=p.notch(3).bw  depth=p.notch(3).depth  gain=1  samplePeriod=samplePeriod
  notch filter 4 : LibControllers/notch filter  SystemSampleTime=-1  freq=p.notch(4).freq  bw=p.notch(4).bw  depth=p.notch(4).depth  gain=1  samplePeriod=samplePeriod
  notch filter 5 : LibControllers/notch filter  SystemSampleTime=-1  freq=p.notch(5).freq  bw=p.notch(5).bw  depth=p.notch(5).depth  gain=1  samplePeriod=samplePeriod
  out : Outport
  wires:
  notch filter 4/1 -> notch filter 5/1
  notch filter 3/1 -> notch filter 4/1
  notch filter 2/1 -> notch filter 3/1
  notch filter 1/1 -> notch filter 2/1
  notch filter 5/1 -> out/1
  inp/1 -> notch filter 1/1
